simulink model "L4Zadatak1"  (R2017a)
settings: Solver=ode45  StartTime=0.0  StopTime=15  RelTol=1e-3  EnableMultiTasking=on
settings Model: Creator=student  LastModifiedBy=korisnik
settings DataIOCC: LimitDataPoints=on  SaveFormat=Array  SignalLoggingSaveFormat=ModelDataLogs
settings OptimizationCC: ExpressionDepthLimit=2147483647  LifeSpan=inf
settings DebuggingCC: UnderspecifiedInitializationDetection=Classic  MergeDetectMultiDrivingBlocksExec=none  SolverPrmCheckMsg=warning  FcnCallInpInsideContextMsg=warning  StateNameClashWarn=warning  SFUnexpectedBacktrackingDiag=warning  SFNoUnconditionalDefaultTransitionDiag=warning  SFExecutionAtInitializationDiag=none
settings HardwareCC: ProdBitPerPointer=32  ProdBitPerSizeT=32  ProdBitPerPtrDiffT=32  ProdLargestAtomicFloat=None  ProdIntDivRoundTo=Undefined  ProdEndianess=Unspecified  ProdWordSize=32  ProdHWDeviceType=32-bit Generic
settings ModelReferenceCC: PropagateSignalLabelsOutOfModel=off
settings GRTTargetCC: TargetLangStandard=C89/C90 (ANSI)  GeneratePreprocessorConditionals=Disable all  CombineOutputUpdateFcns=off  GRTInterface=on
settings ConfigComp: CovMetricSettings=dw  CovHtmlReporting=on  CovSaveCumulativeToWorkspaceVar=on  CovSaveSingleToWorkspaceVar=on  CovExternalEMLEnable=off

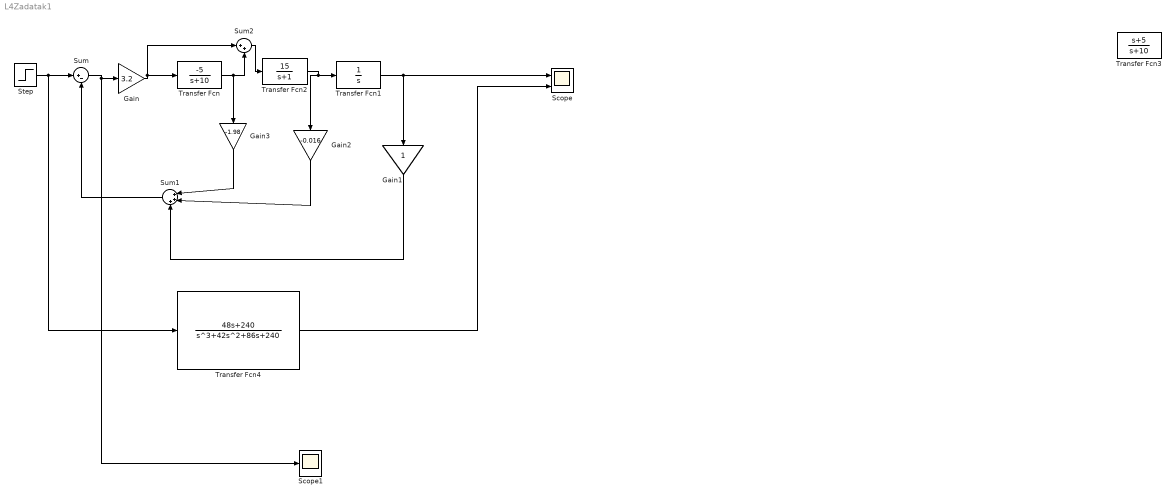
== system L4Zadatak1 ==
  Gain : Gain  Gain=3.2
  Gain1 : Gain
  Gain2 : Gain  Gain=-0.016
  Gain3 : Gain  Gain=-1.98
  Scope : Scope  NumInputPorts=2
  Scope1 : Scope
  Step : Step  SampleTime=0
  Sum : Sum  Inputs=|+-
  Sum1 : Sum  Inputs=|+++
  Sum2 : Sum  Inputs=|++
  Transfer Fcn : TransferFcn  Numerator=[-5]  Denominator=[1 10]
  Transfer Fcn1 : TransferFcn  Denominator=[1 0 ]
  Transfer Fcn2 : TransferFcn  Numerator=[0 15]  Denominator=[1 1]
  Transfer Fcn3 : TransferFcn  Numerator=[1 5]  Denominator=[1 10]
  Transfer Fcn4 : TransferFcn  Numerator=[48 240]  Denominator=[1 42 86 240]
  wires:
  Step/1 -> Sum/1, Transfer Fcn4/1
  Sum/1 -> Scope1/1, Gain/1
  Transfer Fcn/1 -> Sum2/2, Gain3/1
  Transfer Fcn2/1 -> Transfer Fcn1/1, Gain2/1
  Gain3/1 -> Sum1/1
  Transfer Fcn1/1 -> Gain1/1, Scope/1
  Gain1/1 -> Sum1/3
  Gain2/1 -> Sum1/2
  Sum1/1 -> Sum/2
  Gain/1 -> Transfer Fcn/1, Sum2/1
  Transfer Fcn4/1 -> Scope/2
  Sum2/1 -> Transfer Fcn2/1
